simulink model "am_3"  (Simulink 4.00)
settings: Solver=ode45  StartTime=0  StopTime=1  RelTol=1e-3
undefined symbols (not defined in the file or in its folder): B, fn, k
libraries: dsparch3 x5, commsource2 x2, dspstat3 x2, dspmathops x2
Description:
  | Model lacza cyfrowego z modulacja ASK/FSK/PSK
settings Model: Creator=Tomas  LimitDataPoints=off  MaxDataPoints=10000  RTWOptions="-aEnforceIntegerDowncast=1 -aExtMode=0 -aFoldNonRolledExpr=1 -aForceParamTrailComments=0 -aGenerateComments=1 -aIgnoreCustomStorageClasses=1 -aIncHierarchyInIds=0 -aInlineInvariantSignals=0 -aLocalBlockOutputs=1 -aLogVarNameModifier=\"rt_\" -aRTWVerbose=1 -aRollThreshold=5 -aShowEliminatedStatements=1"  RTWInlineParameters=on  BlockReductionOpt=off

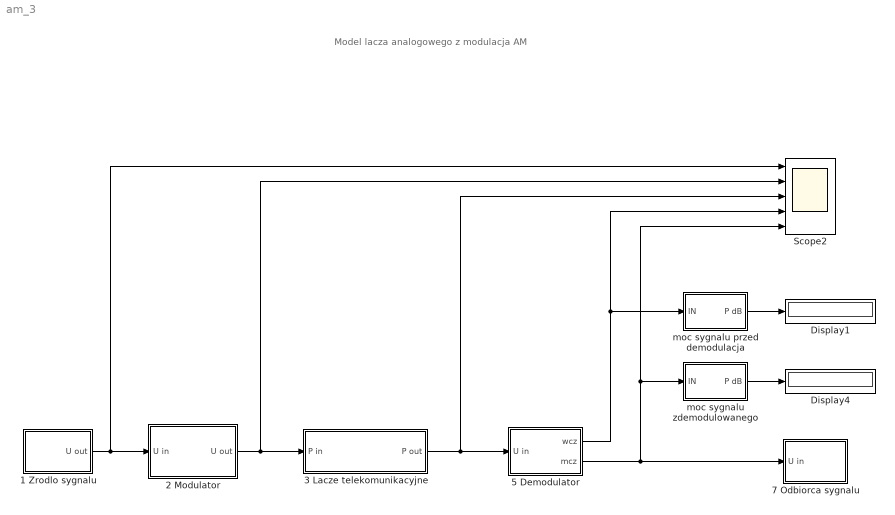
== system am_3 ==
  note: Model lacza analogowego z modulacja AM
  1 Zrodlo sygnalu : Subsystem  mask(Źródło sygnału){on=on, sq=off, bity=300}
      mask prompts: on "Włączenie źródła sygnału"; sq "Przebieg losowy"; bity "częstotliwość/pasmo"
      mask help:
      | Generuje sygnał testowy.
      | Moc wyjściowa -6 dB.
      mask init:
      | if (sq == 0) sq = 1;
      | else sq = 0;
      | end;
      | if (on == 0)
      | set_param(gcb,'MaskEnables',{,'on','off','off'}); fgen=100; G=1;
      | else
      |   set_param(gcb,'MaskEnables',{,'on','on','on'});
      |   if (bity == 1) fgen = 100; G=1/0.1791;
      |   elseif (bity == 2) fgen = 200; G=1/0.2467;
      |   else fgen = 300; G=1/0.3022;
      |   end;
      | end;
      settings: RTWFcnNameOpts=Auto  RTWFileNameOpts=Auto
      mask Help: No help
      mask StyleString: checkbox,checkbox,popup(100|200|300)
      mask Display: disp('Sygnal\nnadawany')
  2 Modulator : Subsystem  mask(Modulator AM){on=off, p=0.7}
      mask prompts: on "Włączenie modulatora"; p "Głębokość modulacji (0..1):"
      mask help:
      | Dokonuje operacji modulacji AM sygnałem podanym na wejście.
      | Częstotliość nośnej: 1000 Hz.
      mask init:
      | fnos=1000;
      | if (on==0) k=1; set_param(gcb,'MaskEnables',{,'on','off'});
      | else set_param(gcb,'MaskEnables',{,'on','on'});
      |   if (p == 1) k = 0.1;
      |   elseif (p == 2) k = 0.2;
      |   elseif (p == 3) k = 0.3;
      |   elseif (p == 4) k = 0.4;
      |   elseif (p == 5) k = 0.5;
      |   elseif (p == 6) k = 0.6;
      |   elseif (p == 7) k = 0.7;
      |   elseif (p == 8) k = 0.8;
      |   elseif (p == 9) k = 0.9;
      |   elseif (p == 10) k = 1.0;
      |   else k = 1.5;
      |   end;
      | end;
      | on=on+1;
      settings: RTWFcnNameOpts=Auto  RTWFileNameOpts=Auto
      mask Help: No help
      mask StyleString: checkbox,popup(0.1|0.2|0.3|0.4|0.5|0.6|0.7|0.8|0.9|1.0|1.5)
      mask Display: disp('Modulator\nAM')
  "3 Lacze telekomunikacyjne " : Subsystem  mask(Łącze telekomunikacyjne){wn=on, sz=3}
      mask prompts: wn "Dodanie szumu białego"; sz "Moc szumu [dB]:"
      mask help:
      | Filtruje i tłumi sygnał wejściowy według zadanych parametrów.
      | Na sygnał nakładany jest też szum biały wg rozkładu Gaussa.
      mask init:
      | sz=10^(sz/10);
      | if (wn == 0)
      | set_param(gcb,'MaskEnables',{,'on','off'});
      | else
      | set_param(gcb,'MaskEnables',{,'on','on'});
      | end;
      settings: RTWFcnNameOpts=Auto  RTWFileNameOpts=Auto
      mask Display: disp('Lacze \ntelekomunikacyjne')
  5 Demodulator : Subsystem  mask(Demodulator AM){typ=detektor obwiedni, on=off, p=200}
      mask prompts: typ "Wybór typu demodulatora"; on "włącz filtr pasmowy"; p "pasmo filtru (Hz)"
      mask help:
      | Dokonuje operacji demodulacji AM sygnału podanego na wejście.
      | Częstotliwość nośnej: 1000 Hz.
      mask init:
      | fn=1000;
      | if (on==0) B=400; set_param(gcb,'MaskEnables',{,'on','on','off'});
      | else set_param(gcb,'MaskEnables',{,'on','on','on'});
      |   if (p == 1) B = 50;
      |   elseif (p == 2) B = 75;
      |   elseif (p == 3) B = 100;
      |   elseif (p == 4) B = 150;
      |   elseif (p == 5) B = 200;
      |   elseif (p == 6) B = 250;
      |   elseif (p == 7) B = 300;
      |   elseif (p == 8) B = 350;
      |   elseif (p == 9) B = 400;
      |   elseif (p == 10) B = 500;
      |   else B = 600;
      |   end;
      | B=16/15*B;
      | end;
      settings: RTWFcnNameOpts=Auto  RTWFileNameOpts=Auto
      mask Help: No help.
      mask StyleString: popup(detektor obwiedni|detektor synchroniczny),checkbox,popup(50|75|100|150|200|250|300|350|400|500|600)
      mask Display: disp('Demodulator\nAM')
  7 Odbiorca sygnalu : Subsystem
      settings: RTWFcnNameOpts=Auto  RTWFileNameOpts=Auto
      mask Type: Odbiorca sygnału
      mask Description: Odbiera sygnał przesylany od nadawcy.
      mask Help: No help
      mask Display: disp('Sygnal\nodbierany')
  Display1 : Display
      settings: Format=short
  Display4 : Display
      settings: Format=short
  Scope2 : Scope  NumInputPorts=5
      settings: TimeRange=1  YMin=-1~-2.5~-2.5~0~-5  YMax=1~2.5~2.5~1.75~5  SaveToWorkspace=off  SaveName=ScopeData  DataFormat=Array  MaxDataPoints=10000
  moc sygnalu zdemodulowanego : Subsystem  mask(Power dB){on=on}
      mask prompts: on "włącz"
      mask help: Oblicza w dB wartość mocy mierzonego sygnału
      settings: RTWFcnNameOpts=Auto  RTWFileNameOpts=Auto
  moc sygnalu przed demodulacja : Subsystem  mask(Power dB){on=on}
      mask prompts: on "włącz"
      mask help: Oblicza w dB wartość mocy mierzonego sygnału
      settings: RTWFcnNameOpts=Auto  RTWFileNameOpts=Auto
  wires:
  1 Zrodlo sygnalu/1(U out) -> 2 Modulator/1(U in), Scope2/1
  5 Demodulator/2(mcz) -> moc sygnalu zdemodulowanego/1(IN), Scope2/5, 7 Odbiorca sygnalu/1(U in)
  2 Modulator/1(U out) -> "3 Lacze telekomunikacyjne "/1(P in), Scope2/2
  "3 Lacze telekomunikacyjne "/1(P out) -> 5 Demodulator/1(U in), Scope2/3
  moc sygnalu zdemodulowanego/1(P dB) -> Display4/1
  5 Demodulator/1(wcz) -> Scope2/4, moc sygnalu przed demodulacja/1(IN)
  moc sygnalu przed demodulacja/1(P dB) -> Display1/1

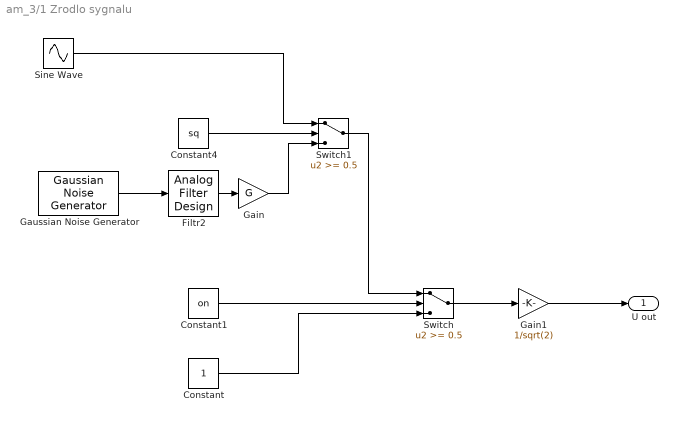
== system am_3/1 Zrodlo sygnalu ==
  Constant : Constant  Value=1
  Constant1 : Constant  Value=on
  Constant4 : Constant  Value=sq
  Filtr2 : dsparch3/Analog Filter Design  method=Chebyshev II  filttype=Lowpass  N=16  Wlo=2*pi*fgen  Whi=2*pi*(fn+B/2)  Rp=2  Rs=60
  Gain : Gain  Gain=G  Multiplication=Element-wise(K.*u)  SaturateOnIntegerOverflow=on
  Gain1 : Gain  Gain=1/sqrt(2)  Multiplication=Element-wise(K.*u)  SaturateOnIntegerOverflow=on
  Gaussian Noise Generator : commsource2/Gaussian Noise Generator  m=0  d=1  s=12345  Ts=1/(6000)  frameBased=off  sampPerFrame=1  orient=off
  Sine Wave : Sin  SineType=Time-based  Amplitude=sqrt(2)  Bias=0  Frequency=2*pi*fgen  Phase=0  Samples=10  SampleTime=0  Offset=0
  Switch : Switch  Threshold=0.5
  Switch1 : Switch  Threshold=0.5
  U out : Outport  Port=1
  wires:
  Switch/1 -> Gain1/1
  Constant1/1 -> Switch/2
  Switch1/1 -> Switch/1
  Constant4/1 -> Switch1/2
  Sine Wave/1 -> Switch1/1
  Constant/1 -> Switch/3
  Gaussian Noise Generator/1 -> Filtr2/1
  Filtr2/1 -> Gain/1
  Gain/1 -> Switch1/3
  Gain1/1 -> U out/1

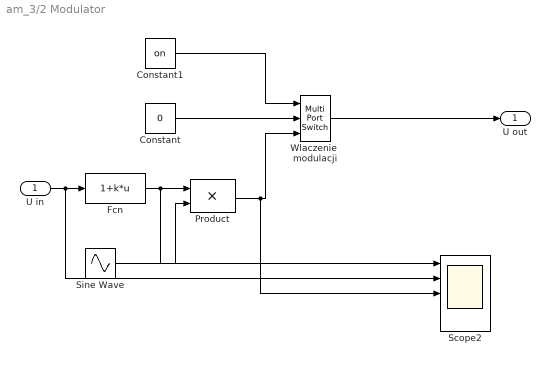
== system am_3/2 Modulator ==
  U in : Inport  Port=1  LatchInput=off
  Constant : Constant  Value=0
  Constant1 : Constant  Value=on
  Fcn : Fcn  Expr=1+k*u
  Product : Product  Inputs=2  Multiplication=Element-wise(.*)  SaturateOnIntegerOverflow=on
  Scope2 : Scope  NumInputPorts=5
      settings: TimeRange=0.4  YMin=-1~-2.5~-2.5~0~-5  YMax=1~2.5~2.5~1.75~5  SaveToWorkspace=off  DataFormat=Array  MaxDataPoints=10000
  Sine Wave : Sin  SineType=Time-based  Amplitude=1  Bias=0  Frequency=2*pi*1000  Phase=0  Samples=10  SampleTime=0  Offset=0
  Wlaczenie  modulacji : MultiPortSwitch  Inputs=2
  U out : Outport  Port=1
  wires:
  Wlaczenie  modulacji/1 -> U out/1
  Constant1/1 -> Wlaczenie  modulacji/1
  Constant/1 -> Wlaczenie  modulacji/2
  Product/1 -> Wlaczenie  modulacji/3, Scope2/3
  U in/1 -> Fcn/1, Scope2/2
  Fcn/1 -> Product/1, Scope2/1
  Sine Wave/1 -> Product/2

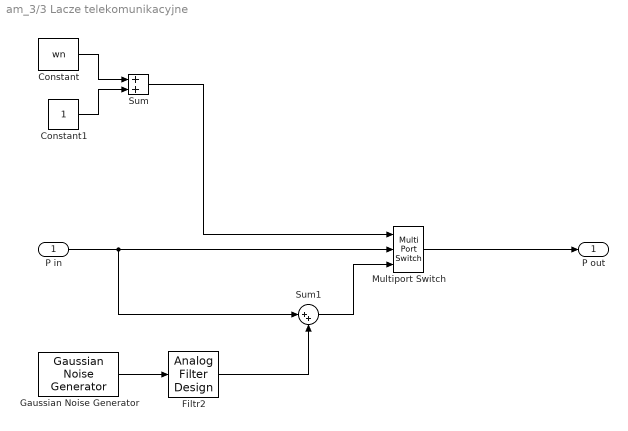
== system am_3/3 Lacze telekomunikacyjne  ==
  P in : Inport  Port=1  LatchInput=off
  Constant : Constant  Value=wn
  Constant1 : Constant  Value=1
  Filtr2 : dsparch3/Analog Filter Design  method=Butterworth  filttype=Lowpass  N=2  Wlo=2*pi*1000  Whi=2*pi*(fn+B/2)  Rp=2  Rs=40
  Gaussian Noise Generator : commsource2/Gaussian Noise Generator  m=0  d=sz/0.7333  s=12345  Ts=1/(6000)  frameBased=off  sampPerFrame=1  orient=off
  Multiport Switch : MultiPortSwitch  Inputs=2
  Sum : Sum  Inputs=++  SaturateOnIntegerOverflow=on
  Sum1 : Sum  Inputs=|++  SaturateOnIntegerOverflow=on
  P out : Outport  Port=1
  wires:
  P in/1 -> Sum1/1, Multiport Switch/2
  Constant/1 -> Sum/1
  Constant1/1 -> Sum/2
  Sum/1 -> Multiport Switch/1
  Multiport Switch/1 -> P out/1
  Sum1/1 -> Multiport Switch/3
  Gaussian Noise Generator/1 -> Filtr2/1
  Filtr2/1 -> Sum1/2

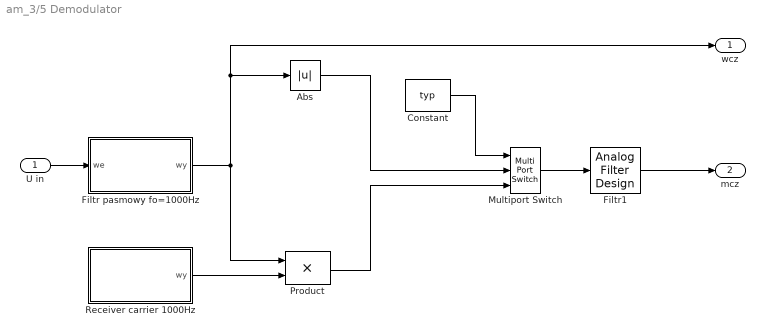
== system am_3/5 Demodulator ==
  U in : Inport  Port=1  LatchInput=off
  Abs : Abs  SaturateOnIntegerOverflow=on
  Constant : Constant  Value=typ
  Filtr pasmowy fo=1000Hz : Subsystem
      settings: RTWFcnNameOpts=Auto  RTWFileNameOpts=Auto
  Filtr1 : dsparch3/Analog Filter Design  method=Chebyshev II  filttype=Lowpass  N=16  Wlo=2*pi*(fn-B/2)  Whi=2*pi*(fn+B/2)  Rp=2  Rs=60
  Multiport Switch : MultiPortSwitch  Inputs=2
  Product : Product  Inputs=2  Multiplication=Element-wise(.*)  SaturateOnIntegerOverflow=on
  Receiver carrier 1000Hz : Subsystem
      settings: RTWFcnNameOpts=Auto  RTWFileNameOpts=Auto
  wcz : Outport  Port=1
  mcz : Outport  Port=2
  wires:
  Multiport Switch/1 -> Filtr1/1
  Abs/1 -> Multiport Switch/2
  Constant/1 -> Multiport Switch/1
  Receiver carrier 1000Hz/1(wy) -> Product/2
  Product/1 -> Multiport Switch/3
  Filtr pasmowy fo=1000Hz/1(wy) -> Product/1, Abs/1, wcz/1
  U in/1 -> Filtr pasmowy fo=1000Hz/1(we)
  Filtr1/1 -> mcz/1

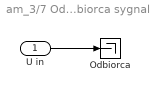
== system am_3/7 Odbiorca sygnalu ==
  U in : Inport  Port=1  LatchInput=off
  Odbiorca : Terminator
  wires:
  U in/1 -> Odbiorca/1

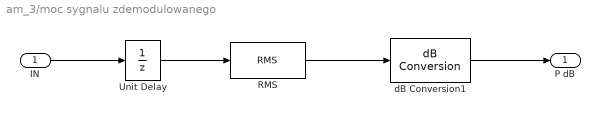
== system am_3/moc sygnalu zdemodulowanego ==
  IN : Inport  Port=1  LatchInput=off
  RMS : dspstat3/RMS  run=on  reset_popup=None
  Unit Delay : UnitDelay  X0=0  SampleTime=1/2048
      settings: RTWStateStorageClass=Auto
  dB Conversion1 : dspmathops/dB Conversion  dBtype=dB  intype=Amplitude  R=1  fuzz=on
  P dB : Outport  Port=1
  wires:
  dB Conversion1/1 -> P dB/1
  RMS/1 -> dB Conversion1/1
  IN/1 -> Unit Delay/1
  Unit Delay/1 -> RMS/1

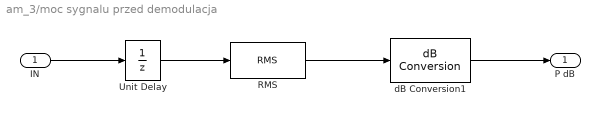
== system am_3/moc sygnalu przed demodulacja ==
  IN : Inport  Port=1  LatchInput=off
  RMS : dspstat3/RMS  run=on  reset_popup=None
  Unit Delay : UnitDelay  X0=0  SampleTime=1/4096
      settings: RTWStateStorageClass=Auto
  dB Conversion1 : dspmathops/dB Conversion  dBtype=dB  intype=Amplitude  R=1  fuzz=on
  P dB : Outport  Port=1
  wires:
  dB Conversion1/1 -> P dB/1
  RMS/1 -> dB Conversion1/1
  IN/1 -> Unit Delay/1
  Unit Delay/1 -> RMS/1

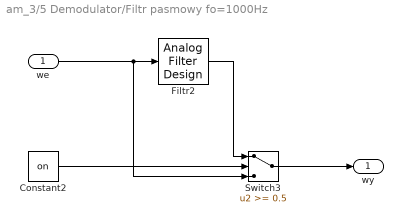
== system am_3/5 Demodulator/Filtr pasmowy fo=1000Hz ==
  we : Inport  Port=1  LatchInput=off
  Constant2 : Constant  Value=on
  Filtr2 : dsparch3/Analog Filter Design  method=Chebyshev II  filttype=Bandpass  N=20  Wlo=2*pi*(fn-B/2)  Whi=2*pi*(fn+B/2)  Rp=2  Rs=60
  Switch3 : Switch  Threshold=0.5
  wy : Outport  Port=1
  wires:
  we/1 -> Filtr2/1, Switch3/3
  Constant2/1 -> Switch3/2
  Filtr2/1 -> Switch3/1
  Switch3/1 -> wy/1

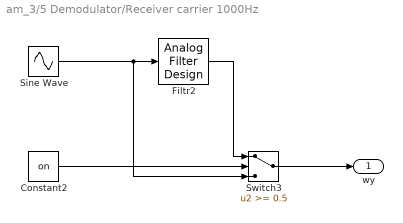
== system am_3/5 Demodulator/Receiver carrier 1000Hz ==
  Constant2 : Constant  Value=on
  Filtr2 : dsparch3/Analog Filter Design  method=Chebyshev II  filttype=Bandpass  N=20  Wlo=2*pi*(fn-B/2)  Whi=2*pi*(fn+B/2)  Rp=2  Rs=60
  Sine Wave : Sin  SineType=Time-based  Amplitude=1  Bias=0  Frequency=2*pi*fn  Phase=0  Samples=10  SampleTime=0  Offset=0
  Switch3 : Switch  Threshold=0.5
  wy : Outport  Port=1
  wires:
  Sine Wave/1 -> Filtr2/1, Switch3/3
  Constant2/1 -> Switch3/2
  Filtr2/1 -> Switch3/1
  Switch3/1 -> wy/1
